simulink model "closed_loop_sim"  (R2024a)
settings: Solver=ode45  StartTime=0.0  StopTime=15.0  MaxStep=0.01  RelTol=1e-3  AbsTol=1e-6
undefined symbols (not defined in the file): K_lat, K_long, X0, X_lat_trim, X_long_trim
settings Model: Creator=mkaarthi  LastModifiedBy=mkaarthi

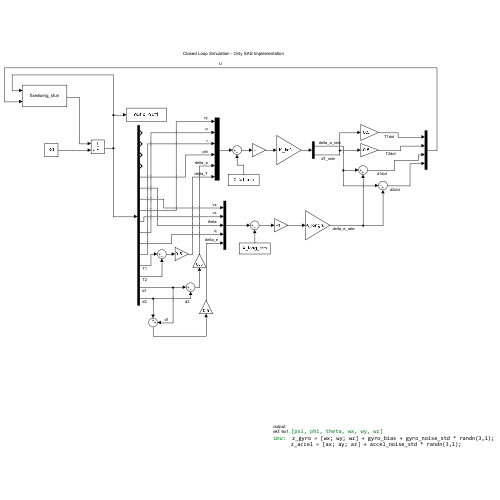
[thumbnail: Simulink's stored preview of the top-level diagram]
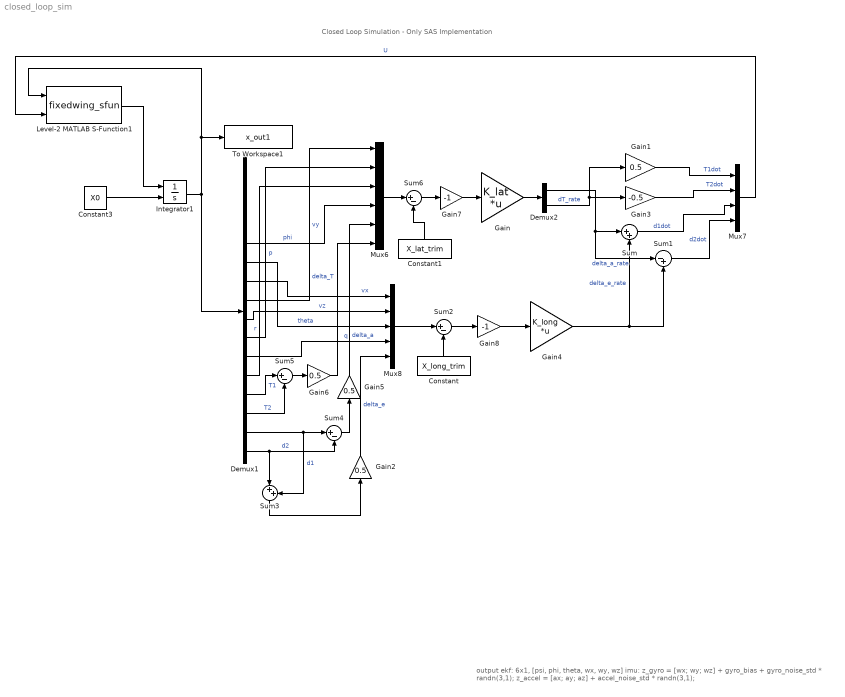
== system closed_loop_sim ==
  note: output
      | ekf: 6x1, [psi, phi, theta, wx, wy, wz]
      | imu: z_gyro = [wx; wy; wz] + gyro_bias + gyro_noise_std * randn(3,1);
      | z_accel = [ax; ay; az] + accel_noise_std * randn(3,1);
  note: Closed Loop Simulation - Only SAS Implementation
  Constant : Constant  Value=X_long_trim
  Constant1 : Constant  Value=X_lat_trim
  Constant3 : Constant  Value=X0
  Demux1 : Demux  Outputs=16
  Demux2 : Demux  Outputs=2
  Gain : Gain  Gain=K_lat  Multiplication=Matrix(K*u)
  Gain{1..2,5..6} (4 alike) : Gain  Gain=0.5
  Gain3 : Gain  Gain=-0.5
  Gain4 : Gain  Gain=K_long  Multiplication=Matrix(K*u)
  Gain7 : Gain  Gain=-1
  Gain8 : Gain  Gain=-1
  Integrator1 : Integrator  InitialConditionSource=external
  Level-2 MATLAB S-Function1 : M-S-Function  FunctionName=fixedwing_sfun
  Mux6 : Mux  Inputs=6
  Mux7 : Mux
  Mux8 : Mux  Inputs=5
  Sum : Sum  Inputs=|++
  Sum1 : Sum  Inputs=|-+
  Sum{2,4..6} (4 alike) : Sum  Inputs=|+-
  Sum3 : Sum  Inputs=|++
  To Workspace1 : ToWorkspace  VariableName=x_out1  SampleTime=-1
  wires:
  Demux1/6 -> Mux8/3  "theta"
  Gain3/1 -> Mux7/2  "T2dot"
  Demux1/10 -> Mux6/2  "p"
  Demux1/11 -> Mux8/4  "q"
  Integrator1/1 -> Demux1/1, To Workspace1/1, Level-2 MATLAB S-Function1/1
  Gain/1 -> Demux2/1
  Demux1/8 -> Mux6/1  "vy"
  Demux1/9 -> Mux8/2  "vz"
  Mux7/1 -> Level-2 MATLAB S-Function1/2  "U"
  Constant3/1 -> Integrator1/2
  Demux1/5 -> Mux6/4  "phi"
  Sum/1 -> Mux7/3  "d1dot"
  Sum1/1 -> Mux7/4  "d2dot"
  Demux2/2 -> Gain1/1, Gain3/1  "dT_rate"
  Gain4/1 -> Sum1/2, Sum/2  "delta_e_rate"
  Demux2/1 -> Sum1/1, Sum/1  "delta_a_rate"
  Gain1/1 -> Mux7/1  "T1dot"
  Demux1/12 -> Mux6/3  "r"
  Demux1/7 -> Mux8/1  "vx"
  Level-2 MATLAB S-Function1/1 -> Integrator1/1
  Mux8/1 -> Sum2/1
  Constant/1 -> Sum2/2
  Demux1/16 -> Sum4/2, Sum3/1  "d2"
  Demux1/15 -> Sum4/1, Sum3/2  "d1"
  Sum3/1 -> Gain2/1
  Sum4/1 -> Gain5/1
  Demux1/13 -> Sum5/1  "T1"
  Demux1/14 -> Sum5/2  "T2"
  Sum5/1 -> Gain6/1
  Gain2/1 -> Mux8/5  "delta_e"
  Gain5/1 -> Mux6/5  "delta_a"
  Gain6/1 -> Mux6/6  "delta_T"
  Sum2/1 -> Gain8/1
  Gain8/1 -> Gain4/1
  Gain7/1 -> Gain/1
  Sum6/1 -> Gain7/1
  Mux6/1 -> Sum6/1
  Constant1/1 -> Sum6/2
